simulink model "HexrotorDynamicModel_2015a_March"  (Simulink 8.5)
settings: Solver=ode3  SolverMode=SingleTasking  StartTime=0.0  StopTime=10  FixedStep=0.001  RelTol=1e-3
values from neighbouring files (symbols this model uses):
  alpha = pi/180 * 13.6    (= 0.237364778271)    [IdealParameter.m]    (also in ParLuk11.m = deg2rad(13.6); Parameter.m = [-alpha_i;alpha_i;-alpha_i;alpha_i;-alpha_i;alpha_i]; ParameterIdeal.m = [-alpha_i;alpha_i;-alpha_i;alpha_i;-alpha_i;alpha_i]; ParameterVIVE.m = [alpha_i;-alpha_i;alpha_i;-alpha_i;alpha_i;-alpha_i])
  alpha_0 = alpha    (= 0.237364778271)    [IdealParameter.m]    (also in Parameter.m = alpha; ParameterIdeal.m = alpha*1.01; ParameterVIVE.m = alpha*1.01; ParameterVO.m = alpha*1.01)
  angular_noise = 0    [IdealParameter.m]    (also in Parameter.m = 0.5; ParameterIdeal.m; ParameterVIVE.m; ParameterVO.m)
  b = 1.1e-06    [IdealParameter.m]    (also in ParLuk11.m = 1.14e-07; Parameter.m = 8.944e-07; ParameterIdeal.m; ParameterVIVE.m)
  b_0 = b*1.15    (= 1.265e-06)    [IdealParameter.m]    (also in Parameter.m = 8.944e-07; ParameterIdeal.m; ParameterVIVE.m; ParameterVO.m)
  beta = 0    [IdealParameter.m]    (also in ParLuk11.m; Parameter.m = [beta_i; beta_i; beta_i; beta_i; beta_i; beta_i]; ParameterIdeal.m = [beta_i; beta_i; beta_i; beta_i; beta_i; beta_i]; ParameterVIVE.m = [beta_i; beta_i; beta_i; beta_i; beta_i; beta_i])
  beta_0 = beta    (= 0)    [IdealParameter.m]    (also in Parameter.m = beta; ParameterIdeal.m = beta*0.99; ParameterVIVE.m = beta*0.99; ParameterVO.m = beta*0.99)
  eta = 1    [Controllability.m]    (also in IdealParameter.m = 75; Parameter.m = 2; ParameterIdeal.m = 40; ParameterVIVE.m = 10)
  eta_rot = 50    [IdealParameter.m]    (also in Parameter.m = 2; ParameterIdeal.m = 20; ParameterVIVE.m = 5; ParameterVO.m = 2)
  g = 9.81    [IdealParameter.m]    (also in ParLuk11.m; Parameter.m; ParameterIdeal.m; ParameterVIVE.m)
  g_0 = g*0.99    (= 9.7119)    [IdealParameter.m]    (also in Parameter.m = 9.81; ParameterIdeal.m = 9.81; ParameterVIVE.m = 9.81; ParameterVO.m = 9.81)
  IB = [Ixx 0 0; 0 Iyy 0; 0 0 Izz]    [IdealParameter.m]    (also in ParLuk11.m; Parameter.m; ParameterIdeal.m; ParameterVIVE.m)
  IB_0 = IB*1.07    [IdealParameter.m]    (also in Parameter.m = IB; ParameterIdeal.m; ParameterVIVE.m; ParameterVO.m)
  k = 5.6e-05    [IdealParameter.m]    (also in ParLuk11.m = 2.98e-06; Parameter.m = 4.472e-05; ParameterIdeal.m; ParameterVIVE.m = 5.13e-05)
  K_0 = Ts/(T_rotor_0+Ts)    (= 0.0384615384615)    [IdealParameter.m]    (also in Parameter.m = 0.230769230769; ParameterIdeal.m; ParameterVIVE.m = 0.0350877192982; ParameterVO.m = 0.214285714286)
  k_0 = k*1.16    (= 6.496e-05)    [IdealParameter.m]    (also in Parameter.m = 4.472e-05; ParameterIdeal.m; ParameterVIVE.m = 5.9508e-05; ParameterVO.m)
  K_d = diag([5,5,5,2,2,2])    [ParLuk11.m]
  K_p1 = 10*eye(3)    [ParLuk11.m]
  k_p2 = 3    [ParLuk11.m]
  K_P_1 = 15*eye(3)    [IdealParameter.m]    (also in Parameter.m = 2*eye(3); ParameterIdeal.m; ParameterVIVE.m = 10*eye(3); ParameterVO.m = 2*eye(3))
  K_P_2 = 50*eye(3)    [IdealParameter.m]    (also in Parameter.m = 4*eye(3); ParameterIdeal.m; ParameterVIVE.m = 10*eye(3); ParameterVO.m = 4*eye(3))
  K_P_3 = 60*eye(3)    [IdealParameter.m]    (also in Parameter.m = 6*eye(3); ParameterIdeal.m; ParameterVIVE.m = 10*eye(3); ParameterVO.m = 6*eye(3))
  K_P_D = 30*eye(3)    [IdealParameter.m]    (also in ParLuk11.m = 10*eye(3); Parameter.m = 5*eye(3); ParameterIdeal.m; ParameterVIVE.m = 15*eye(3))
  K_P_I = 100*eye(3)    [IdealParameter.m]    (also in ParLuk11.m = 10*eye(3); Parameter.m = 10*eye(3); ParameterIdeal.m = 80*eye(3); ParameterVIVE.m)
  K_P_P = 100*eye(3)    [IdealParameter.m]    (also in ParLuk11.m = 20*eye(3); Parameter.m = 10*eye(3); ParameterIdeal.m = 130*eye(3); ParameterVIVE.m)
  K_R_1 = 40*eye(3)    [IdealParameter.m]    (also in Parameter.m = 2*eye(3); ParameterIdeal.m; ParameterVIVE.m = 10*eye(3); ParameterVO.m = 2*eye(3))
  K_R_2 = 100*eye(3)    [IdealParameter.m]    (also in Parameter.m = 4*eye(3); ParameterIdeal.m; ParameterVIVE.m = 10*eye(3); ParameterVO.m = 4*eye(3))
  K_R_3 = 50*eye(4)    [IdealParameter.m]    (also in Parameter.m = 6*eye(4); ParameterIdeal.m; ParameterVIVE.m = 10*eye(4); ParameterVO.m = 6*eye(4))
  K_R_D = 30*eye(3)    [IdealParameter.m]    (also in ParLuk11.m = 10*eye(3); Parameter.m = 5*eye(3); ParameterIdeal.m; ParameterVIVE.m = 15*eye(3))
  K_R_I = 100*eye(3)    [IdealParameter.m]    (also in ParLuk11.m = 10*eye(3); Parameter.m = 10*eye(3); ParameterIdeal.m = 80*eye(3); ParameterVIVE.m)
  K_R_P = 100*eye(3)    [IdealParameter.m]    (also in ParLuk11.m = 20*eye(3); Parameter.m = 10*eye(3); ParameterIdeal.m = 130*eye(3); ParameterVIVE.m)
  L = 0.4    [IdealParameter.m]    (also in ParLuk11.m = 1; Parameter.m; ParameterIdeal.m; ParameterVIVE.m = 0.6)
  L_0 = L*1.02    (= 0.408)    [IdealParameter.m]    (also in Parameter.m = 0.4; ParameterIdeal.m; ParameterVIVE.m = 0.612; ParameterVO.m)
  lambda = 10    [IdealParameter.m]    (also in Parameter.m = 3; ParameterIdeal.m = 5; ParameterVIVE.m = 5; ParameterVO.m = 3)
  lambda_rot = 10    [IdealParameter.m]    (also in Parameter.m = 3; ParameterIdeal.m; ParameterVIVE.m = 5; ParameterVO.m = 3)
  m = 1    [Controllability.m]    (also in IdealParameter.m = 2.5; ParLuk11.m = 0.6; Parameter.m = 4.85; ParameterIdeal.m = 4.85)
  M = 50    [IdealParameter.m]    (also in Parameter.m = 6; ParameterIdeal.m = 100; ParameterVIVE.m = 5; ParameterVO.m = 6)
  m_0 = m*1.03    (= 2.575)    [IdealParameter.m]    (also in Parameter.m = 4.85; ParameterIdeal.m = 4.9955; ParameterVIVE.m = 4.52994; ParameterVO.m = 4.9955)
  M_rot = 50    [IdealParameter.m]    (also in Parameter.m = 6; ParameterIdeal.m = 15; ParameterVIVE.m = 1; ParameterVO.m = 6)
  omega_noise = 0    [IdealParameter.m]    (also in Parameter.m = sqrt(2)*angular_noise/Ts * pi/180; ParameterIdeal.m; ParameterVIVE.m; ParameterVO.m)
  p_noise = 0    [IdealParameter.m]    (also in Parameter.m = 0.001; ParameterIdeal.m; ParameterVIVE.m; ParameterVO.m)
  T_delay = 0    [IdealParameter.m]    (also in Parameter.m = 0.1; ParameterIdeal.m; ParameterVIVE.m = 0.04; ParameterVO.m = 0.1)
  T_rotor = 0.1    [IdealParameter.m]    (also in Parameter.m; ParameterIdeal.m; ParameterVIVE.m; ParameterVO.m)
  Ts = 1/250    (= 0.004)    [IdealParameter.m]    (also in Parameter.m = 0.03; ParameterIdeal.m; ParameterVIVE.m; ParameterVO.m = 0.03)
  v_noise = 0    [IdealParameter.m]    (also in Parameter.m = sqrt(2)*p_noise/Ts; ParameterIdeal.m; ParameterVIVE.m; ParameterVO.m)
  z_p_0 = T_rotor_0/(T_rotor_0+Ts)    (= 0.961538461538)    [IdealParameter.m]    (also in Parameter.m = 0.769230769231; ParameterIdeal.m; ParameterVIVE.m = 0.964912280702; ParameterVO.m = 0.785714285714)
undefined symbols (not defined in the file or in its folder): DiscIntNeverNeededParam, k_ad, k_ap, k_pd, k_pp, k_z
libraries: vrlib x9, simulink x7, dspmtrx3 x3
(part 3 of 3)

== matlab function Backstepping1/MATLAB Function1 ==
  data: R input double; q output double
function q   = DCM2Quat(R)

%%%%%%%%%%%%%%%%%%%%%%%%%%%%%%%%%%%%%%%%%%%%%%%%%%%%%%%%%%%%%%%%%%%%%%%%%%%
%
% M-file: Tool_DCM2Quat
%         -> impelmeted as M-Function
% Author: Marcel Tkocz
% Version: 27.01.2008
%
% Description:
%   This Function converts roll-pitch-yaw angels into their quaternion
%   equivalents.
%
% Inputs:
%   Orientation ... orientation in roll-pitch-yaw angels
%
% Outputs:
%   q           ... orientation in quaternions
%   
%%%%%%%%%%%%%%%%%%%%%%%%%%%%%%%%%%%%%%%%%%%%%%%%%%%%%%%%%%%%%%%%%%%%%%%%%%%

%--------------------------------------------------------------------------
% Calculation of Quaternions based on q1
%--------------------------------------------------------------------------
q = [0 0 0 1]';

if (1 + R(1,1) - R(2,2) - R(3,3)) > 0 
    q1 = 1/2*sqrt(1 + R(1,1) - R(2,2) - R(3,3));
    q2 = 1/(4*q1)*( R(1,2) + R(2,1));
    q3 = 1/(4*q1)*( R(1,3) + R(3,1));
    q4 = 1/(4*q1)*(-R(2,3) + R(3,2));

    if round(q1) ~= 0
        q = [q1; q2; q3; q4];
    end
end

%--------------------------------------------------------------------------
% Calculation of Quaternions based on q2
%--------------------------------------------------------------------------

if (1 - R(1,1) + R(2,2) - R(3,3)) > 0
    q2 = 1/2*sqrt(1 - R(1,1) + R(2,2) - R(3,3));
    q1 = 1/(4*q2)*( R(1,2) + R(2,1));
    q3 = 1/(4*q2)*( R(2,3) + R(3,2));
    q4 = 1/(4*q2)*( R(1,3) - R(3,1));

    if round(q2) ~= 0
        q = [q1; q2; q3; q4];
    end
end

%--------------------------------------------------------------------------
% Calculation of Quaternions based on q3
%--------------------------------------------------------------------------

if (1 - R(1,1) - R(2,2) + R(3,3)) > 0
    q3 = 1/2*sqrt(1 - R(1,1) - R(2,2) + R(3,3));
    q1 = 1/(4*q3)*( R(1,3) + R(3,1));
    q2 = 1/(4*q3)*( R(2,3) + R(3,2));
    q4 = 1/(4*q3)*(-R(1,2) + R(2,1));

    if round(q3) ~= 0
        q = [q1; q2; q3; q4];
    end
end

%--------------------------------------------------------------------------
% Calculation of Quaternions based on q4
%--------------------------------------------------------------------------

if (1 + R(1,1) + R(2,2) + R(3,3)) > 0
    q4 = 1/2*sqrt(1 + R(1,1) + R(2,2) + R(3,3));
    q1 = 1/(4*q4)*(-R(2,3) + R(3,2));
    q2 = 1/(4*q4)*(-R(3,1) + R(1,3));
    q3 = 1/(4*q4)*(-R(1,2) + R(2,1));

    if round(q4) ~= 0
        q = [q1; q2; q3; q4];
    end
end


end

== matlab function Backstepping1/MATLAB Function2 ==
  data: eta_tilde input double; z1 output double; eps_tilde input double
function z1 = compute_z1(eta_tilde, eps_tilde)

z1 = [1-abs(eta_tilde);
    eps_tilde];

== matlab function Backstepping1/MATLAB Function3 ==
  data: eta_tilde input double; G output double; eps_tilde input double
function G = compute_G(eta_tilde, eps_tilde)

if (eta_tilde >= 0)
    sig = 1;
else
    sig = -1;
end

G = [sig*eps_tilde';
    eye(3)*eta_tilde + vec2skew(eps_tilde)]';

== matlab function Backstepping1/MATLAB Function4 ==
  data: K1 input double; alpha_dot output double; G input double; z1 input double; z2 input double; omega_tilde input double; eta_tilde input double; eps_tilde input double
function alpha_dot = compute_alpha_dot(K1,G,z1,z2, omega_tilde, eta_tilde, eps_tilde)

eta_dot = -0.5*eps_tilde'*omega_tilde;

eps_dot = 0.5*(eta_tilde*eye(3) + vec2skew(eps_tilde))*omega_tilde;

if eta_tilde >= 0
    sig = 1;
else
    sig = -1;
end

G_dot = [sig*eps_dot';
        eta_dot*eye(3) + vec2skew(eps_dot)]';

% alpha_dot = -K1 ( G_dot * z1 + G * z1_dot)
alpha_dot = -K1*(G_dot*z1  + G*(-0.5*G'*K1*G*z1 + 0.5*G'*z2));

== matlab function Backstepping1/MATLAB Function5 ==
  data: J input double; J_inv output double
function J_inv = inverse(J)

J_inv = inv(J);

== matlab function Backstepping1/MATLAB Function6 ==
  data: R_m input double; JR output double; I_B input double
function JR = computeJR(R_m, I_B)
JR = [R_m zeros(3);
     zeros(3) inv(I_B) ];

== matlab function Backstepping1/MATLAB Function7 ==
  data: R input double; q output double
function q   = DCM2Quat(R)

%%%%%%%%%%%%%%%%%%%%%%%%%%%%%%%%%%%%%%%%%%%%%%%%%%%%%%%%%%%%%%%%%%%%%%%%%%%
%
% M-file: Tool_DCM2Quat
%         -> impelmeted as M-Function
% Author: Marcel Tkocz
% Version: 27.01.2008
%
% Description:
%   This Function converts roll-pitch-yaw angels into their quaternion
%   equivalents.
%
% Inputs:
%   Orientation ... orientation in roll-pitch-yaw angels
%
% Outputs:
%   q           ... orientation in quaternions
%   
%%%%%%%%%%%%%%%%%%%%%%%%%%%%%%%%%%%%%%%%%%%%%%%%%%%%%%%%%%%%%%%%%%%%%%%%%%%

%--------------------------------------------------------------------------
% Calculation of Quaternions based on q1
%--------------------------------------------------------------------------
q = [0 0 0 1]';

if (1 + R(1,1) - R(2,2) - R(3,3)) > 0 
    q1 = 1/2*sqrt(1 + R(1,1) - R(2,2) - R(3,3));
    q2 = 1/(4*q1)*( R(1,2) + R(2,1));
    q3 = 1/(4*q1)*( R(1,3) + R(3,1));
    q4 = 1/(4*q1)*(-R(2,3) + R(3,2));

    if round(q1) ~= 0
        q = [q1; q2; q3; q4];
    end
end

%--------------------------------------------------------------------------
% Calculation of Quaternions based on q2
%--------------------------------------------------------------------------

if (1 - R(1,1) + R(2,2) - R(3,3)) > 0
    q2 = 1/2*sqrt(1 - R(1,1) + R(2,2) - R(3,3));
    q1 = 1/(4*q2)*( R(1,2) + R(2,1));
    q3 = 1/(4*q2)*( R(2,3) + R(3,2));
    q4 = 1/(4*q2)*( R(1,3) - R(3,1));

    if round(q2) ~= 0
        q = [q1; q2; q3; q4];
    end
end

%--------------------------------------------------------------------------
% Calculation of Quaternions based on q3
%--------------------------------------------------------------------------

if (1 - R(1,1) - R(2,2) + R(3,3)) > 0
    q3 = 1/2*sqrt(1 - R(1,1) - R(2,2) + R(3,3));
    q1 = 1/(4*q3)*( R(1,3) + R(3,1));
    q2 = 1/(4*q3)*( R(2,3) + R(3,2));
    q4 = 1/(4*q3)*(-R(1,2) + R(2,1));

    if round(q3) ~= 0
        q = [q1; q2; q3; q4];
    end
end

%--------------------------------------------------------------------------
% Calculation of Quaternions based on q4
%--------------------------------------------------------------------------

if (1 + R(1,1) + R(2,2) + R(3,3)) > 0
    q4 = 1/2*sqrt(1 + R(1,1) + R(2,2) + R(3,3));
    q1 = 1/(4*q4)*(-R(2,3) + R(3,2));
    q2 = 1/(4*q4)*(-R(3,1) + R(1,3));
    q3 = 1/(4*q4)*(-R(1,2) + R(2,1));

    if round(q4) ~= 0
        q = [q1; q2; q3; q4];
    end
end


end

== matlab function Backstepping1/MATLAB Function8 ==
  data: I input double; I_inv output double
function I_inv = inverse(I)

I_inv = inv(I);

== matlab function Integral Backstepping/MATLAB Function9 ==
  data: K1 input double; alpha output double; G input double; z1 input double; K3 input double; Xsi input double
function alpha = compute_alpha(K1,G,z1,K3,Xsi)

%alpha = -K1*G*z1 - 2*pinv(G.')*K3*Xsi;
alpha = -K1*G*z1 - 2*G*K3*Xsi;

== matlab function Zero Moment Control [Mic17] unfertig/MATLAB Function9 ==
  data: R input double; q output double
function q   = DCM2Quat(R)

%%%%%%%%%%%%%%%%%%%%%%%%%%%%%%%%%%%%%%%%%%%%%%%%%%%%%%%%%%%%%%%%%%%%%%%%%%%
%
% M-file: Tool_DCM2Quat
%         -> impelmeted as M-Function
% Author: Marcel Tkocz
% Version: 27.01.2008
%
% Description:
%   This Function converts roll-pitch-yaw angels into their quaternion
%   equivalents.
%
% Inputs:
%   Orientation ... orientation in roll-pitch-yaw angels
%
% Outputs:
%   q           ... orientation in quaternions
%   
%%%%%%%%%%%%%%%%%%%%%%%%%%%%%%%%%%%%%%%%%%%%%%%%%%%%%%%%%%%%%%%%%%%%%%%%%%%

%--------------------------------------------------------------------------
% Calculation of Quaternions based on q1
%--------------------------------------------------------------------------
q = [0 0 0 1]';

if (1 + R(1,1) - R(2,2) - R(3,3)) > 0 
    q1 = 1/2*sqrt(1 + R(1,1) - R(2,2) - R(3,3));
    q2 = 1/(4*q1)*( R(1,2) + R(2,1));
    q3 = 1/(4*q1)*( R(1,3) + R(3,1));
    q4 = 1/(4*q1)*(-R(2,3) + R(3,2));

    if round(q1) ~= 0
        q = [q1; q2; q3; q4];
    end
end

%--------------------------------------------------------------------------
% Calculation of Quaternions based on q2
%--------------------------------------------------------------------------

if (1 - R(1,1) + R(2,2) - R(3,3)) > 0
    q2 = 1/2*sqrt(1 - R(1,1) + R(2,2) - R(3,3));
    q1 = 1/(4*q2)*( R(1,2) + R(2,1));
    q3 = 1/(4*q2)*( R(2,3) + R(3,2));
    q4 = 1/(4*q2)*( R(1,3) - R(3,1));

    if round(q2) ~= 0
        q = [q1; q2; q3; q4];
    end
end

%--------------------------------------------------------------------------
% Calculation of Quaternions based on q3
%--------------------------------------------------------------------------

if (1 - R(1,1) - R(2,2) + R(3,3)) > 0
    q3 = 1/2*sqrt(1 - R(1,1) - R(2,2) + R(3,3));
    q1 = 1/(4*q3)*( R(1,3) + R(3,1));
    q2 = 1/(4*q3)*( R(2,3) + R(3,2));
    q4 = 1/(4*q3)*(-R(1,2) + R(2,1));

    if round(q3) ~= 0
        q = [q1; q2; q3; q4];
    end
end

%--------------------------------------------------------------------------
% Calculation of Quaternions based on q4
%--------------------------------------------------------------------------

if (1 + R(1,1) + R(2,2) + R(3,3)) > 0
    q4 = 1/2*sqrt(1 + R(1,1) + R(2,2) + R(3,3));
    q1 = 1/(4*q4)*(-R(2,3) + R(3,2));
    q2 = 1/(4*q4)*(-R(3,1) + R(1,3));
    q3 = 1/(4*q4)*(-R(1,2) + R(2,1));

    if round(q4) ~= 0
        q = [q1; q2; q3; q4];
    end
end


end

== matlab function Geometric Control on SE(3) [Ras17]/MATLAB Function9 ==
  data: K_P1 input double; WI output double; H_er input double; kp2 input double
function WI = computeWI(K_P1, H_er, kp2)
R_er = H_er(1:3,1:3);
eta_er = H_er(1:3,4);

%phi = 0.5*trace(K_P1*(eye(3)-R_er)) + 0.5*abs(kp2)+ norm(eta_er)^2;
%WI = -[1,1,1,1,1,1]'*phi;

WI = -kp2*[0;0;0;eta_er];

== matlab function Sliding Mode Control/MATLAB Function1 ==
  data: R input double; q output double
function q   = DCM2Quat(R)

%%%%%%%%%%%%%%%%%%%%%%%%%%%%%%%%%%%%%%%%%%%%%%%%%%%%%%%%%%%%%%%%%%%%%%%%%%%
%
% M-file: Tool_DCM2Quat
%         -> impelmeted as M-Function
% Author: Marcel Tkocz
% Version: 27.01.2008
%
% Description:
%   This Function converts roll-pitch-yaw angels into their quaternion
%   equivalents.
%
% Inputs:
%   Orientation ... orientation in roll-pitch-yaw angels
%
% Outputs:
%   q           ... orientation in quaternions
%   
%%%%%%%%%%%%%%%%%%%%%%%%%%%%%%%%%%%%%%%%%%%%%%%%%%%%%%%%%%%%%%%%%%%%%%%%%%%

%--------------------------------------------------------------------------
% Calculation of Quaternions based on q1
%--------------------------------------------------------------------------
q = [0 0 0 1]';

if (1 + R(1,1) - R(2,2) - R(3,3)) > 0 
    q1 = 1/2*sqrt(1 + R(1,1) - R(2,2) - R(3,3));
    q2 = 1/(4*q1)*( R(1,2) + R(2,1));
    q3 = 1/(4*q1)*( R(1,3) + R(3,1));
    q4 = 1/(4*q1)*(-R(2,3) + R(3,2));

    if round(q1) ~= 0
        q = [q1; q2; q3; q4];
    end
end

%--------------------------------------------------------------------------
% Calculation of Quaternions based on q2
%--------------------------------------------------------------------------

if (1 - R(1,1) + R(2,2) - R(3,3)) > 0
    q2 = 1/2*sqrt(1 - R(1,1) + R(2,2) - R(3,3));
    q1 = 1/(4*q2)*( R(1,2) + R(2,1));
    q3 = 1/(4*q2)*( R(2,3) + R(3,2));
    q4 = 1/(4*q2)*( R(1,3) - R(3,1));

    if round(q2) ~= 0
        q = [q1; q2; q3; q4];
    end
end

%--------------------------------------------------------------------------
% Calculation of Quaternions based on q3
%--------------------------------------------------------------------------

if (1 - R(1,1) - R(2,2) + R(3,3)) > 0
    q3 = 1/2*sqrt(1 - R(1,1) - R(2,2) + R(3,3));
    q1 = 1/(4*q3)*( R(1,3) + R(3,1));
    q2 = 1/(4*q3)*( R(2,3) + R(3,2));
    q4 = 1/(4*q3)*(-R(1,2) + R(2,1));

    if round(q3) ~= 0
        q = [q1; q2; q3; q4];
    end
end

%--------------------------------------------------------------------------
% Calculation of Quaternions based on q4
%--------------------------------------------------------------------------

if (1 + R(1,1) + R(2,2) + R(3,3)) > 0
    q4 = 1/2*sqrt(1 + R(1,1) + R(2,2) + R(3,3));
    q1 = 1/(4*q4)*(-R(2,3) + R(3,2));
    q2 = 1/(4*q4)*(-R(3,1) + R(1,3));
    q3 = 1/(4*q4)*(-R(1,2) + R(2,1));

    if round(q4) ~= 0
        q = [q1; q2; q3; q4];
    end
end


end

== matlab function Sliding Mode Control/MATLAB Function7 ==
  data: R input double; q output double
function q   = DCM2Quat(R)

%%%%%%%%%%%%%%%%%%%%%%%%%%%%%%%%%%%%%%%%%%%%%%%%%%%%%%%%%%%%%%%%%%%%%%%%%%%
%
% M-file: Tool_DCM2Quat
%         -> impelmeted as M-Function
% Author: Marcel Tkocz
% Version: 27.01.2008
%
% Description:
%   This Function converts roll-pitch-yaw angels into their quaternion
%   equivalents.
%
% Inputs:
%   Orientation ... orientation in roll-pitch-yaw angels
%
% Outputs:
%   q           ... orientation in quaternions
%   
%%%%%%%%%%%%%%%%%%%%%%%%%%%%%%%%%%%%%%%%%%%%%%%%%%%%%%%%%%%%%%%%%%%%%%%%%%%

%--------------------------------------------------------------------------
% Calculation of Quaternions based on q1
%--------------------------------------------------------------------------
q = [0 0 0 1]';

if (1 + R(1,1) - R(2,2) - R(3,3)) > 0 
    q1 = 1/2*sqrt(1 + R(1,1) - R(2,2) - R(3,3));
    q2 = 1/(4*q1)*( R(1,2) + R(2,1));
    q3 = 1/(4*q1)*( R(1,3) + R(3,1));
    q4 = 1/(4*q1)*(-R(2,3) + R(3,2));

    if round(q1) ~= 0
        q = [q1; q2; q3; q4];
    end
end

%--------------------------------------------------------------------------
% Calculation of Quaternions based on q2
%--------------------------------------------------------------------------

if (1 - R(1,1) + R(2,2) - R(3,3)) > 0
    q2 = 1/2*sqrt(1 - R(1,1) + R(2,2) - R(3,3));
    q1 = 1/(4*q2)*( R(1,2) + R(2,1));
    q3 = 1/(4*q2)*( R(2,3) + R(3,2));
    q4 = 1/(4*q2)*( R(1,3) - R(3,1));

    if round(q2) ~= 0
        q = [q1; q2; q3; q4];
    end
end

%--------------------------------------------------------------------------
% Calculation of Quaternions based on q3
%--------------------------------------------------------------------------

if (1 - R(1,1) - R(2,2) + R(3,3)) > 0
    q3 = 1/2*sqrt(1 - R(1,1) - R(2,2) + R(3,3));
    q1 = 1/(4*q3)*( R(1,3) + R(3,1));
    q2 = 1/(4*q3)*( R(2,3) + R(3,2));
    q4 = 1/(4*q3)*(-R(1,2) + R(2,1));

    if round(q3) ~= 0
        q = [q1; q2; q3; q4];
    end
end

%--------------------------------------------------------------------------
% Calculation of Quaternions based on q4
%--------------------------------------------------------------------------

if (1 + R(1,1) + R(2,2) + R(3,3)) > 0
    q4 = 1/2*sqrt(1 + R(1,1) + R(2,2) + R(3,3));
    q1 = 1/(4*q4)*(-R(2,3) + R(3,2));
    q2 = 1/(4*q4)*(-R(3,1) + R(1,3));
    q3 = 1/(4*q4)*(-R(1,2) + R(2,1));

    if round(q4) ~= 0
        q = [q1; q2; q3; q4];
    end
end


end

== matlab function Sliding Mode Control/MATLAB Function ==
  data: s input double; u output double; z2 input double; p_dotdot_d input double; g input double; lambda input double; eta input double
function u = computeU(s,z2,p_dotdot_d,g,lambda,eta)

sgn = zeros(3,1);
% avoid chattering
% linear function
% for it=1:3
%     if s(it) < 1 && s(it) > -1
%         sgn(it) = s(it);
%     else
%         sgn(it) = sign(s(it));
%     end
% end
% smoother atan function
sgn = 2/pi*atan(s);
u = -lambda*z2 + g + p_dotdot_d - eta*sgn;

== matlab function Sliding Mode Control/MATLAB Function5 ==
  data: J input double; J_inv output double
function J_inv = inverse(J)

J_inv = inv(J);

== matlab function Sliding Mode Control/MATLAB Function6 ==
  data: R_m input double; JR output double; I_B input double
function JR = computeJR(R_m, I_B)
JR = [R_m zeros(3);
     zeros(3) inv(I_B) ];

== matlab function Sliding Mode Control/MATLAB Function2 ==
  data: I input double; I_inv output double
function I_inv = inverse(I)

I_inv = inv(I);

== matlab function Sliding Mode Control/MATLAB Function3 ==
  data: epsilon_d input double; eta_d input double; epsilon input double; eta input double; eta_tilde output double; epsilon_tilde output double; epsilon_tilde_T output double; skew_eps_tilde output double
function [eta_tilde, epsilon_tilde, epsilon_tilde_T, skew_eps_tilde] = calc_q_tilde(epsilon_d, eta_d, epsilon, eta)

eta_tilde = eta_d*eta + epsilon_d'*epsilon;

epsilon_tilde = -eta * epsilon_d + eta_d*epsilon - vec2skew(epsilon_d)*epsilon;

epsilon_tilde_T = epsilon_tilde';

skew_eps_tilde = vec2skew(epsilon_tilde);

== matlab function Sliding Mode Control/MATLAB Function4 ==
  data: eta_tilde input double; z1 output double; eps_tilde input double
function z1 = compute_z1(eta_tilde, eps_tilde)

z1 = [1-abs(eta_tilde);
    eps_tilde];

== matlab function Sliding Mode Control/MATLAB Function8 ==
  data: eta_tilde input double; G output double; eps_tilde input double
function G = compute_G(eta_tilde, eps_tilde)

if (eta_tilde >= 0)
    sig = 1;
else
    sig = -1;
end

G = [sig*eps_tilde';
    eye(3)*eta_tilde + vec2skew(eps_tilde)]';

== matlab function Sliding Mode Control/MATLAB Function9 ==
  data: G input double; z2 output double; omega_tilde input double
function z2 = compute_z2(G,omega_tilde)

z2 = 0.5*G.'*omega_tilde;

== matlab function Sliding Mode Control/MATLAB Function10 ==
  data: eps_tilde input double; G_dot output double; eta_tilde input double; omega_tilde input double
function G_dot = compute_G_dot(eps_tilde, eta_tilde, omega_tilde)

eta_dot = -0.5*eps_tilde'*omega_tilde;

eps_dot = 0.5*(eta_tilde*eye(3) + vec2skew(eps_tilde))*omega_tilde;

if eta_tilde >= 0
    sig = 1;
else
    sig = -1;
end

G_dot = [sig*eps_dot';
        eta_dot*eye(3) + vec2skew(eps_dot)]';

== matlab function Sliding Mode Control/MATLAB Function11 ==
  data: s input double; u output double; z2 input double; lambda input double; G input double; G_dot input double; omega_tilde input double; omega_d_dot input double; omega_B input double; IBB input double; eta input double
function u = compute_u(s,z2,lambda,G,G_dot,omega_tilde,omega_d_dot,omega_B,IBB,eta)

sgn = zeros(4,1);
% avoid chattering
% linear function
for it=1:4
%     if s(it) < 1 && s(it) > -1
%         sgn(it) = s(it);
%     else
%         sgn(it) = sign(s(it));
%     end
    sgn(it) = 2/pi*atan(s(it));
end

u = IBB*G* ( -2*eta*sgn - 2*lambda*z2 - G_dot.'*omega_tilde ) ...
    + IBB*omega_d_dot + cross(omega_B,IBB*omega_B);

== matlab function compute nominal Coupling Matrices/MATLAB Function5 ==
  data: e_r1 output double; e_r2 output double; e_r3 output double; e_r4 output double; e_r5 output double; e_r6 output double; alpha input double; beta input double
function [e_r1, e_r2, e_r3, e_r4, e_r5, e_r6] = computeThrustDirections(alpha, beta)

e_r = zeros(3,6);
for it = 1:6
    alpha_i = alpha *(-1)^(it+1);
    beta_i = beta * (-1)^(it+1);
    gamma_i = (it-1)*pi/3;
    ca = cos(alpha_i);
    sa = sin(alpha_i);
    cb = cos(beta_i);
    sb = sin(beta_i);
    cy = cos(gamma_i);
    sy = sin(gamma_i);
    
    e_r(:,it) = [ca*sb*cy + sa*sy;
                ca*sb*sy - sa*cy;
                ca*cb];
            
end

e_r1 = e_r(:,1);
e_r2 = e_r(:,2);
e_r3 = e_r(:,3);
e_r4 = e_r(:,4);
e_r5 = e_r(:,5);
e_r6 = e_r(:,6);

== matlab function compute nominal Coupling Matrices/MATLAB Function6 ==
  data: F output double; e_r1 input double; e_r2 input double; e_r3 input double; e_r4 input double; e_r5 input double; e_r6 input double; b input double; k input double; L input double; H output double
function [F,H]= computeCouplingMatrix(e_r1, e_r2, e_r3, e_r4, e_r5, e_r6, b, k, L)
% u = w^2

F = zeros(3,6);
H = zeros(3,6);

e_r = [e_r1 e_r2 e_r3 e_r4 e_r5 e_r6];

for it = 1:6
    gamma_i = (it-1)*pi/3;
   
    % thrust direction
    e_ri = e_r(:,it);
    
    % rotor position vector
    r_Ti =  L * [cos(gamma_i);
            sin(gamma_i);
            0];
        
    % Thrust force
    F(:,it) = k*e_ri;   
    
    % thrust and drag moment
    H(:,it) = k * cross(r_Ti, e_ri) + b * (-1)^it * e_ri;
    

    
end

== matlab function Sliding Mode Control/MATLAB Function12 ==
  data: s_0 input double; int_arg output double; eta input double
function int_arg = computeIntArg(s_0,eta)

sgn = 2/pi*atan(s_0);
int_arg = - eta*sgn;

== matlab function Sliding Mode Control/MATLAB Function13 ==
  data: s input double; u1 output double; M input double
function u1 = computeU1(s,M)

sgn = 2/pi*atan(s);
u1 = -M*sgn;%s./norm(s,2);

== matlab function Sliding Mode Control/MATLAB Function14 ==
  data: s_0 input double; int_arg output double; eta input double
function int_arg = computeIntArg(s_0,eta)

sgn = 2/pi*atan(s_0);
int_arg = - eta*sgn;

== matlab function Sliding Mode Control/MATLAB Function15 ==
  data: s input double; G input double; IB input double; u1 output double; M input double
function u1 = computeU1(s,G,IB,M)


D = 0.5*G.'*inv(IB);
u1 = -M*2/pi*atan(D.'*s);%./norm(D.'*s,2);

== matlab function Integral Backstepping Continous /MATLAB Function ==
  data: epsilon_d input double; eta_d input double; epsilon input double; eta input double; eta_tilde output double; epsilon_tilde output double; epsilon_tilde_T output double; skew_eps_tilde output double
function [eta_tilde, epsilon_tilde, epsilon_tilde_T, skew_eps_tilde] = calc_q_tilde(epsilon_d, eta_d, epsilon, eta)

eta_tilde = eta_d*eta + epsilon_d'*epsilon;

epsilon_tilde = eta_d * epsilon - eta*epsilon_d - vec2skew(epsilon_d)*epsilon;

epsilon_tilde_T = epsilon_tilde';

skew_eps_tilde = vec2skew(epsilon_tilde);

== matlab function Integral Backstepping Continous /MATLAB Function1 ==
  data: R input double; q output double
function q   = DCM2Quat(R)

%%%%%%%%%%%%%%%%%%%%%%%%%%%%%%%%%%%%%%%%%%%%%%%%%%%%%%%%%%%%%%%%%%%%%%%%%%%
%
% M-file: Tool_DCM2Quat
%         -> impelmeted as M-Function
% Author: Marcel Tkocz
% Version: 27.01.2008
%
% Description:
%   This Function converts roll-pitch-yaw angels into their quaternion
%   equivalents.
%
% Inputs:
%   Orientation ... orientation in roll-pitch-yaw angels
%
% Outputs:
%   q           ... orientation in quaternions
%   
%%%%%%%%%%%%%%%%%%%%%%%%%%%%%%%%%%%%%%%%%%%%%%%%%%%%%%%%%%%%%%%%%%%%%%%%%%%

%--------------------------------------------------------------------------
% Calculation of Quaternions based on q1
%--------------------------------------------------------------------------
q = [0 0 0 1]';

if (1 + R(1,1) - R(2,2) - R(3,3)) > 0 
    q1 = 1/2*sqrt(1 + R(1,1) - R(2,2) - R(3,3));
    q2 = 1/(4*q1)*( R(1,2) + R(2,1));
    q3 = 1/(4*q1)*( R(1,3) + R(3,1));
    q4 = 1/(4*q1)*(-R(2,3) + R(3,2));

    if round(q1) ~= 0
        q = [q1; q2; q3; q4];
    end
end

%--------------------------------------------------------------------------
% Calculation of Quaternions based on q2
%--------------------------------------------------------------------------

if (1 - R(1,1) + R(2,2) - R(3,3)) > 0
    q2 = 1/2*sqrt(1 - R(1,1) + R(2,2) - R(3,3));
    q1 = 1/(4*q2)*( R(1,2) + R(2,1));
    q3 = 1/(4*q2)*( R(2,3) + R(3,2));
    q4 = 1/(4*q2)*( R(1,3) - R(3,1));

    if round(q2) ~= 0
        q = [q1; q2; q3; q4];
    end
end

%--------------------------------------------------------------------------
% Calculation of Quaternions based on q3
%--------------------------------------------------------------------------

if (1 - R(1,1) - R(2,2) + R(3,3)) > 0
    q3 = 1/2*sqrt(1 - R(1,1) - R(2,2) + R(3,3));
    q1 = 1/(4*q3)*( R(1,3) + R(3,1));
    q2 = 1/(4*q3)*( R(2,3) + R(3,2));
    q4 = 1/(4*q3)*(-R(1,2) + R(2,1));

    if round(q3) ~= 0
        q = [q1; q2; q3; q4];
    end
end

%--------------------------------------------------------------------------
% Calculation of Quaternions based on q4
%--------------------------------------------------------------------------

if (1 + R(1,1) + R(2,2) + R(3,3)) > 0
    q4 = 1/2*sqrt(1 + R(1,1) + R(2,2) + R(3,3));
    q1 = 1/(4*q4)*(-R(2,3) + R(3,2));
    q2 = 1/(4*q4)*(-R(3,1) + R(1,3));
    q3 = 1/(4*q4)*(-R(1,2) + R(2,1));

    if round(q4) ~= 0
        q = [q1; q2; q3; q4];
    end
end


end

== matlab function Integral Backstepping Continous /MATLAB Function2 ==
  data: eta_tilde input double; z1 output double; eps_tilde input double
function z1 = compute_z1(eta_tilde, eps_tilde)

z1 = [1-abs(eta_tilde);
    eps_tilde];

== matlab function Integral Backstepping Continous /MATLAB Function3 ==
  data: eta_tilde input double; G output double; eps_tilde input double
function G = compute_G(eta_tilde, eps_tilde)

if (eta_tilde >= 0)
    sig = 1;
else
    sig = -1;
end

G = [sig*eps_tilde';
    eye(3)*eta_tilde + vec2skew(eps_tilde)]';

== matlab function Integral Backstepping Continous /MATLAB Function4 ==
  data: K1 input double; alpha_dot output double; G input double; z1 input double; z2 input double; omega_tilde input double; eta_tilde input double; eps_tilde input double; K3 input double; Xsi input double
function alpha_dot  = compute_alpha_dot(K1,G,z1,z2, omega_tilde, eta_tilde, eps_tilde, K3, Xsi)

eta_dot = -0.5*eps_tilde'*omega_tilde;

eps_dot = 0.5*(eta_tilde*eye(3) + vec2skew(eps_tilde))*omega_tilde;

if eta_tilde >= 0
    sig = 1;
else
    sig = -1;
end

G_dot = [sig*eps_dot';
        eta_dot*eye(3) + vec2skew(eps_dot)]';

% alpha_dot = -K1 ( G_dot * z1 + G * z1_dot) 
% - 2 (-inv(GT)G_dot inv(GT) * K3 * Xsi + inv(GT)K3*z1
%alpha_dot1 = -K1*(G_dot*z1  + G*(-0.5*G'*K1*G*z1 + 0.5*G'*z2));
alpha_dot1 = -K1*(G_dot*z1  + G*(0.5*G.'*omega_tilde));

%alpha_dot2 = -2*(-pGT*(G_dot.')*pGT*K3*Xsi + pGT*K3*z1);
alpha_dot2 = -2*(G_dot*K3*Xsi + G*K3*z1);
alpha_dot=alpha_dot1+ alpha_dot2;

== matlab function Integral Backstepping Continous /MATLAB Function5 ==
  data: J input double; J_inv output double
function J_inv = inverse(J)

J_inv = inv(J);

== matlab function Integral Backstepping Continous /MATLAB Function6 ==
  data: R_m input double; JR output double; I_B input double
function JR = computeJR(R_m, I_B)
JR = [R_m zeros(3);
     zeros(3) inv(I_B) ];

== matlab function Integral Backstepping Continous /MATLAB Function7 ==
  data: R input double; q output double
function q   = DCM2Quat(R)

%%%%%%%%%%%%%%%%%%%%%%%%%%%%%%%%%%%%%%%%%%%%%%%%%%%%%%%%%%%%%%%%%%%%%%%%%%%
%
% M-file: Tool_DCM2Quat
%         -> impelmeted as M-Function
% Author: Marcel Tkocz
% Version: 27.01.2008
%
% Description:
%   This Function converts roll-pitch-yaw angels into their quaternion
%   equivalents.
%
% Inputs:
%   Orientation ... orientation in roll-pitch-yaw angels
%
% Outputs:
%   q           ... orientation in quaternions
%   
%%%%%%%%%%%%%%%%%%%%%%%%%%%%%%%%%%%%%%%%%%%%%%%%%%%%%%%%%%%%%%%%%%%%%%%%%%%

%--------------------------------------------------------------------------
% Calculation of Quaternions based on q1
%--------------------------------------------------------------------------
q = [0 0 0 1]';

if (1 + R(1,1) - R(2,2) - R(3,3)) > 0 
    q1 = 1/2*sqrt(1 + R(1,1) - R(2,2) - R(3,3));
    q2 = 1/(4*q1)*( R(1,2) + R(2,1));
    q3 = 1/(4*q1)*( R(1,3) + R(3,1));
    q4 = 1/(4*q1)*(-R(2,3) + R(3,2));

    if round(q1) ~= 0
        q = [q1; q2; q3; q4];
    end
end

%--------------------------------------------------------------------------
% Calculation of Quaternions based on q2
%--------------------------------------------------------------------------

if (1 - R(1,1) + R(2,2) - R(3,3)) > 0
    q2 = 1/2*sqrt(1 - R(1,1) + R(2,2) - R(3,3));
    q1 = 1/(4*q2)*( R(1,2) + R(2,1));
    q3 = 1/(4*q2)*( R(2,3) + R(3,2));
    q4 = 1/(4*q2)*( R(1,3) - R(3,1));

    if round(q2) ~= 0
        q = [q1; q2; q3; q4];
    end
end

%--------------------------------------------------------------------------
% Calculation of Quaternions based on q3
%--------------------------------------------------------------------------

if (1 - R(1,1) - R(2,2) + R(3,3)) > 0
    q3 = 1/2*sqrt(1 - R(1,1) - R(2,2) + R(3,3));
    q1 = 1/(4*q3)*( R(1,3) + R(3,1));
    q2 = 1/(4*q3)*( R(2,3) + R(3,2));
    q4 = 1/(4*q3)*(-R(1,2) + R(2,1));

    if round(q3) ~= 0
        q = [q1; q2; q3; q4];
    end
end

%--------------------------------------------------------------------------
% Calculation of Quaternions based on q4
%--------------------------------------------------------------------------

if (1 + R(1,1) + R(2,2) + R(3,3)) > 0
    q4 = 1/2*sqrt(1 + R(1,1) + R(2,2) + R(3,3));
    q1 = 1/(4*q4)*(-R(2,3) + R(3,2));
    q2 = 1/(4*q4)*(-R(3,1) + R(1,3));
    q3 = 1/(4*q4)*(-R(1,2) + R(2,1));

    if round(q4) ~= 0
        q = [q1; q2; q3; q4];
    end
end


end

== matlab function Integral Backstepping Continous /MATLAB Function8 ==
  data: I input double; I_inv output double
function I_inv = inverse(I)

I_inv = inv(I);

== matlab function Integral Backstepping Continous /MATLAB Function9 ==
  data: K1 input double; alpha output double; G input double; z1 input double; K3 input double; Xsi input double
function alpha = compute_alpha(K1,G,z1,K3,Xsi)

%alpha = -K1*G*z1 - 2*pinv(G.')*K3*Xsi;
alpha = -K1*G*z1 - 2*G*K3*Xsi;

== matlab function MATLAB Function1 ==
  data: R input double; eul output double
function eul = DCM2Euler(R)

%Roll
phi = atan2d(R(3,2),R(3,3));

%Pitch
psi = atan2d(-R(3,1),sqrt(R(1,1)^2 + R(2,1)^2));

%Yaw
gamma = atan2d(R(2,1),R(1,1));

eul=[phi;psi;gamma];

== matlab function MATLAB Function ==
  data: rpy input double; R output double
function R = Euler2DCM(rpy)
alpha = rpy(1);
beta = rpy(2);
gamma = rpy(3);

cg = cosd(gamma);
cb = cosd(beta);
sg = sind(gamma);
sb = sind(beta);
sa = sind(alpha);
ca = cosd(alpha);

R = [cg*cb, cg*sb*sa-sg*ca, cg*sb*ca+sg*sa;
    sg*cb, sg*sb*sa+cg*ca, sg*sb*ca-cg*sa;
    -sb, cb*sa, cb*ca];

== matlab function DC Motor Dynamics /MATLAB Function4 ==
  data: u input double; y output double
function y = fcn(u)

y = sqrt(abs(u))*sign(u);

== matlab function DC Motor Dynamics /MATLAB Function5 ==
  data: u input double; y output double
function y = fcn(u)

y = sqrt(abs(u))*sign(u);

== matlab function DC Motor Dynamics /MATLAB Function6 ==
  data: u input double; y output double
function y = fcn(u)

y = u^2*sign(u);
